simulink library "csc_act_actuator_manager_mtv_lib"  (R2014b)
settings: Solver=ode45  StartTime=0.0  StopTime=10.0  RelTol=1e-3
undefined symbols (not defined in the file or in its folder): est_time_step
libraries: csc_vlm_valve_manager_lib x1, csu_ftc_final_thruster_cmd_mtv_lib x1, util_info_lib x1, csu_taf_thruster_arm_fire_mtv_lib x1, csu_tcm_thruster_command_metering_mtv_ib x1
settings Model: Creator=ianmga  LastModifiedBy=mstewart

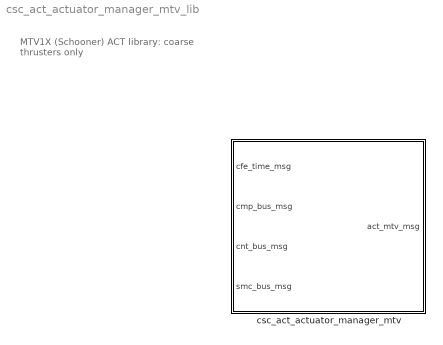
== system csc_act_actuator_manager_mtv_lib ==
  note: MTV1X (Schooner) ACT library:
      | coarse thrusters only
  csc_act_actuator_manager_mtv : Subsystem  Tag=OFSW; MDL_TICK=CNT_BUS_MSG  TreatAsAtomicUnit=on  SystemSampleTime=est_time_step

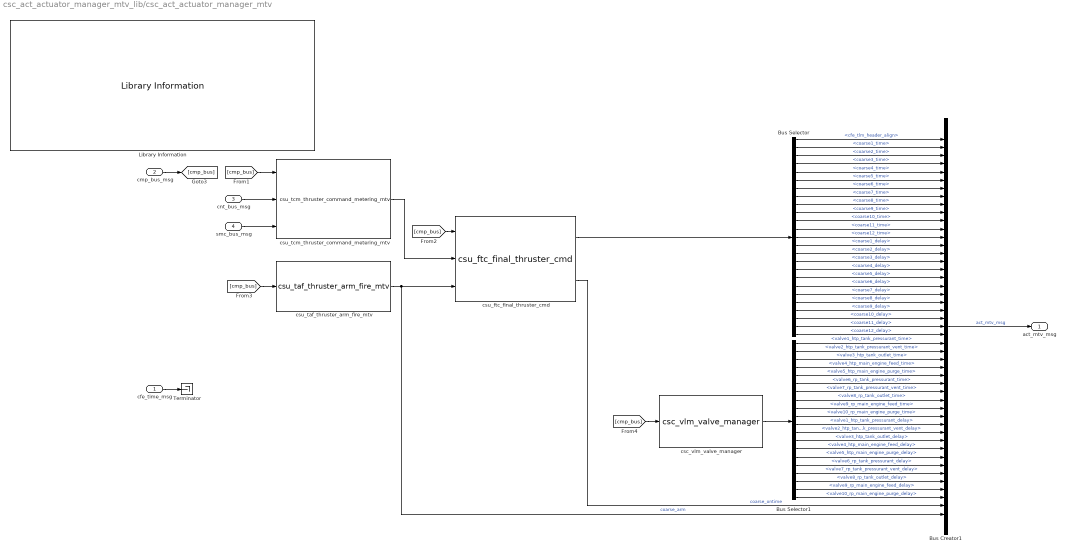
== system csc_act_actuator_manager_mtv_lib/csc_act_actuator_manager_mtv ==
  cfe_time_msg : Inport  OutDataTypeStr=Bus: cfe_time_msg
  cmp_bus_msg : Inport  Port=2
  cnt_bus_msg : Inport  Port=3  OutDataTypeStr=Bus: cnt_bus_msg
  smc_bus_msg : Inport  Port=4
  " csc_vlm_valve_manager" : csc_vlm_valve_manager_lib/ csc_vlm_valve_manager
  " csu_ftc_final_thruster_cmd" : csu_ftc_final_thruster_cmd_mtv_lib/ csu_ftc_final_thruster_cmd
  Bus Creator1 : BusCreator  Inputs=47  OutDataTypeStr=Bus: act_mtv_msg  NonVirtualBus=on
  Bus Selector : BusSelector  OutputSignals=cfe_tlm_header_align,coarse1_time,coarse2_time,coarse3_time,coarse4_time,coarse5_time,coarse6_time,coarse7_time,coarse8_time,coarse9_time,coarse10_time,coarse11_time,coarse12_time,coarse1_delay,coarse2_delay,coarse3_delay,coarse4_delay,coarse5_delay,coarse6_delay,coarse7_delay,coarse8_delay,coarse9_delay,coarse10_delay,coarse11_delay,coarse12_delay
  Bus Selector1 : BusSelector  OutputSignals=valve1_htp_tank_pressurant_time,valve2_htp_tank_pressurant_vent_time,valve3_htp_tank_outlet_time,valve4_htp_main_engine_feed_time,valve5_htp_main_engine_purge_time,valve6_rp_tank_pressurant_time,valve7_rp_tank_pressurant_vent_time,valve8_rp_tank_outlet_time,valve9_rp_main_engine_feed_time,valve10_rp_main_engine_purge_time,valve1_htp_tank_pressurant_delay,valve2_htp_tank_pressurant_vent_delay,valve3_htp_tank_outlet_delay,valve4_htp_main_engine_feed_delay,valve5_htp_main_engine_purge_delay,valve6_rp_tank_pressurant_delay,valve7_rp_tank_pressurant_vent_delay,valve8_rp_tank_outlet_delay,valve9_rp_main_engine_feed_delay,valve10_rp_main_engine_purge_delay
  Library Information : util_info_lib/Library Information  owner='escrane'
  Terminator : Terminator
  csu_taf_thruster_arm_fire_mtv : csu_taf_thruster_arm_fire_mtv_lib/csu_taf_thruster_arm_fire_mtv
  csu_tcm_thruster_command_metering_mtv : csu_tcm_thruster_command_metering_mtv_ib/csu_tcm_thruster_command_metering_mtv
  act_mtv_msg : Outport
  wires:
  Bus Selector/22 -> Bus Creator1/22  "<coarse9_delay>"
  Bus Selector/21 -> Bus Creator1/21  "<coarse8_delay>"
  Bus Selector/20 -> Bus Creator1/20  "<coarse7_delay>"
  Bus Selector/19 -> Bus Creator1/19  "<coarse6_delay>"
  Bus Selector/25 -> Bus Creator1/25  "<coarse12_delay>"
  Bus Selector/14 -> Bus Creator1/14  "<coarse1_delay>"
  Bus Selector/16 -> Bus Creator1/16  "<coarse3_delay>"
  Bus Selector1/20 -> Bus Creator1/45  "<valve10_rp_main_engine_purge_delay>"
  Bus Selector1/19 -> Bus Creator1/44  "<valve9_rp_main_engine_feed_delay>"
  Bus Selector1/18 -> Bus Creator1/43  "<valve8_rp_tank_outlet_delay>"
  Bus Selector1/17 -> Bus Creator1/42  "<valve7_rp_tank_pressurant_vent_delay>"
  Bus Selector1/16 -> Bus Creator1/41  "<valve6_rp_tank_pressurant_delay>"
  Bus Selector1/15 -> Bus Creator1/40  "<valve5_htp_main_engine_purge_delay>"
  Bus Selector1/14 -> Bus Creator1/39  "<valve4_htp_main_engine_feed_delay>"
  Bus Selector1/13 -> Bus Creator1/38  "<valve3_htp_tank_outlet_delay>"
  Bus Selector1/12 -> Bus Creator1/37  "<valve2_htp_tank_pressurant_vent_delay>"
  Bus Selector1/11 -> Bus Creator1/36  "<valve1_htp_tank_pressurant_delay>"
  Bus Selector1/10 -> Bus Creator1/35  "<valve10_rp_main_engine_purge_time>"
  Bus Selector1/9 -> Bus Creator1/34  "<valve9_rp_main_engine_feed_time>"
  Bus Selector1/8 -> Bus Creator1/33  "<valve8_rp_tank_outlet_time>"
  Bus Selector1/7 -> Bus Creator1/32  "<valve7_rp_tank_pressurant_vent_time>"
  Bus Selector1/6 -> Bus Creator1/31  "<valve6_rp_tank_pressurant_time>"
  Bus Selector1/4 -> Bus Creator1/29  "<valve4_htp_main_engine_feed_time>"
  Bus Selector1/3 -> Bus Creator1/28  "<valve3_htp_tank_outlet_time>"
  Bus Selector1/2 -> Bus Creator1/27  "<valve2_htp_tank_pressurant_vent_time>"
  Bus Selector1/1 -> Bus Creator1/26  "<valve1_htp_tank_pressurant_time>"
  Bus Selector1/5 -> Bus Creator1/30  "<valve5_htp_main_engine_purge_time>"
  Bus Creator1/1 -> act_mtv_msg/1  "act_mtv_msg"
  [cmp_bus] -> csu_taf_thruster_arm_fire_mtv/1
  csu_taf_thruster_arm_fire_mtv/1 -> " csu_ftc_final_thruster_cmd"/3, Bus Creator1/47  "coarse_arm"
  " csu_ftc_final_thruster_cmd"/2 -> Bus Creator1/46  "coarse_ontime"
  " csu_ftc_final_thruster_cmd"/1 -> Bus Selector/1
  cfe_time_msg/1 -> Terminator/1
  csu_tcm_thruster_command_metering_mtv/1 -> " csu_ftc_final_thruster_cmd"/2
  cmp_bus_msg/1 -> [cmp_bus]
  [cmp_bus] -> csu_tcm_thruster_command_metering_mtv/1
  [cmp_bus] -> " csu_ftc_final_thruster_cmd"/1
  cnt_bus_msg/1 -> csu_tcm_thruster_command_metering_mtv/2
  smc_bus_msg/1 -> csu_tcm_thruster_command_metering_mtv/3
  [cmp_bus] -> " csc_vlm_valve_manager"/1
  " csc_vlm_valve_manager"/1 -> Bus Selector1/1
  Bus Selector/1 -> Bus Creator1/1  "<cfe_tlm_header_align>"
  Bus Selector/2 -> Bus Creator1/2  "<coarse1_time>"
  Bus Selector/3 -> Bus Creator1/3  "<coarse2_time>"
  Bus Selector/4 -> Bus Creator1/4  "<coarse3_time>"
  Bus Selector/5 -> Bus Creator1/5  "<coarse4_time>"
  Bus Selector/6 -> Bus Creator1/6  "<coarse5_time>"
  Bus Selector/7 -> Bus Creator1/7  "<coarse6_time>"
  Bus Selector/8 -> Bus Creator1/8  "<coarse7_time>"
  Bus Selector/9 -> Bus Creator1/9  "<coarse8_time>"
  Bus Selector/10 -> Bus Creator1/10  "<coarse9_time>"
  Bus Selector/11 -> Bus Creator1/11  "<coarse10_time>"
  Bus Selector/12 -> Bus Creator1/12  "<coarse11_time>"
  Bus Selector/13 -> Bus Creator1/13  "<coarse12_time>"
  Bus Selector/15 -> Bus Creator1/15  "<coarse2_delay>"
  Bus Selector/17 -> Bus Creator1/17  "<coarse4_delay>"
  Bus Selector/18 -> Bus Creator1/18  "<coarse5_delay>"
  Bus Selector/23 -> Bus Creator1/23  "<coarse10_delay>"
  Bus Selector/24 -> Bus Creator1/24  "<coarse11_delay>"
